simulink model "ac_generator_sysid_R2018a"  (R2018a)
settings: Solver=ode15s  StartTime=0.0  StopTime=12  MaxStep=1e-3  RelTol=1e-3
values from neighbouring files (symbols this model uses):
  f_gen = (1-eff)*P/w_g/w_g    (= 4.2217159851)    [ac_generator_parameters.m]
  h = 0.2    [Apollo_LM_design_discrete_observer.m]    (also in Apollo_LM_design_observer.m = 0.25)
  J_gen = 150    [ac_generator_parameters.m]
  K_gen = P/w_g/sind(30)    [ac_generator_parameters.m]
  w_g = 60*2*pi    (= 376.991118431)    [ac_generator_parameters.m]
undefined symbols (not defined in the file or in its folder): den, num
settings Model: Creator=kjartan  LastModifiedBy=kjartan
settings DataIOCC: ReturnWorkspaceOutputs=on
settings DebuggingCC: UnconnectedInputMsg=none  UnconnectedOutputMsg=none  UnconnectedLineMsg=none  SFMachineParentedDataDiag=error
settings ModelReferenceCC: EnableRefExpFcnMdlSchedulingChecks=off
settings SFSimCC: SimUseLocalCustomCode=on
settings RTWCC: Description=Generic Real-Time Target  RTWUseLocalCustomCode=on

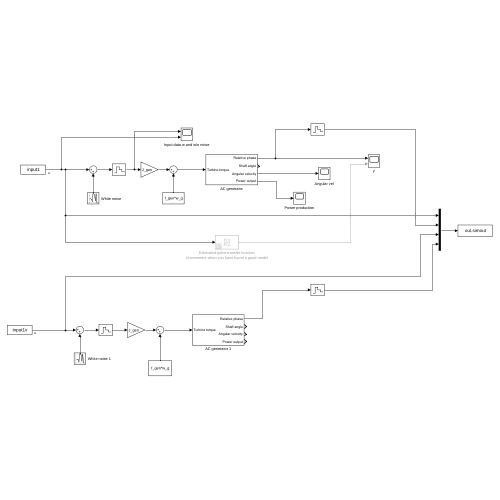
[thumbnail: Simulink's stored preview of the top-level diagram]
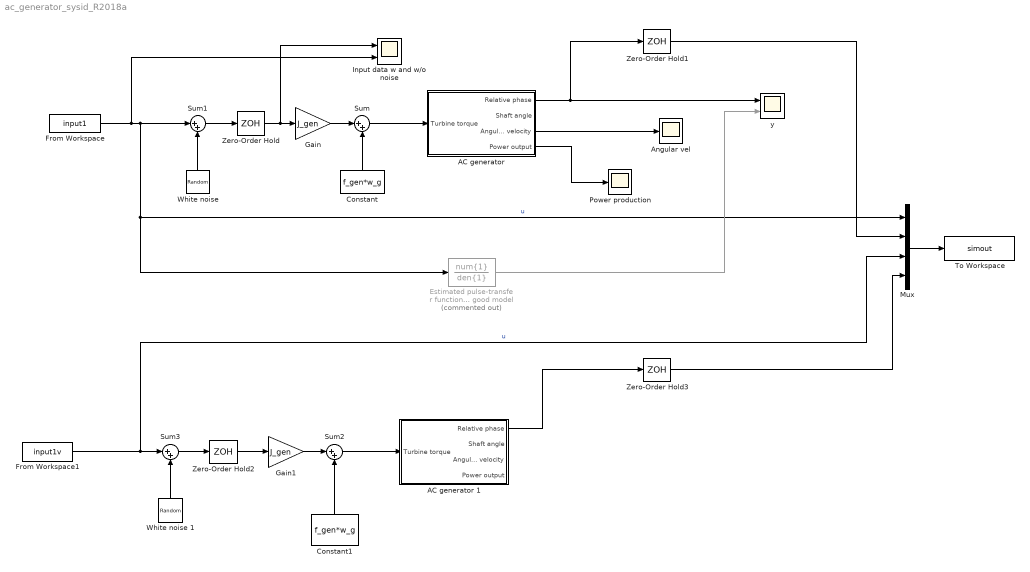
== system ac_generator_sysid_R2018a ==
  AC generator : Subsystem
  AC generator 1 : Subsystem
  Angular vel : Scope
  Constant : Constant  Value=f_gen*w_g
  Constant1 : Constant  Value=f_gen*w_g
  Estimated pulse-transfer function Uncomment when you have found a good model : DiscreteTransferFcn  Commented=on  Numerator=num{1}  Denominator=den{1}  SampleTime=h
  From Workspace : FromWorkspace  VariableName=input1  SampleTime=h
  From Workspace1 : FromWorkspace  VariableName=input1v  SampleTime=h
  Gain : Gain  Gain=J_gen
  Gain1 : Gain  Gain=J_gen
  Input data w and w/o noise : Scope  NumInputPorts=2
  Mux : Mux
  Power production : Scope
  Sum{,1..3} (4 alike) : Sum  Inputs=|++
  To Workspace : ToWorkspace  VariableName=simout  SaveFormat=Timeseries  SampleTime=-1
  White noise : RandomNumber  Variance=0.25  SampleTime=h
  White noise 1 : RandomNumber  Variance=0.25  Seed=9  SampleTime=h
  Zero-Order Hold{,1..3} (4 alike) : ZeroOrderHold  SampleTime=h
  y : Scope  NumInputPorts=2
  wires:
  AC generator/1(Relative phase) -> Zero-Order Hold1/1, y/1
  From Workspace/1 -> Input data w and w/o noise/2, Estimated pulse-transfer function Uncomment when you have found a good model/1, Mux/1, Sum1/1  "u"
  AC generator/3(Angular velocity) -> Angular vel/1
  AC generator/4(Power output) -> Power production/1
  Constant/1 -> Sum/2
  Sum/1 -> AC generator/1(Turbine torque)
  Gain/1 -> Sum/1
  Estimated pulse-transfer function Uncomment when you have found a good model/1 -> y/2
  Zero-Order Hold/1 -> Input data w and w/o noise/1, Gain/1
  Mux/1 -> To Workspace/1
  Zero-Order Hold1/1 -> Mux/2
  Sum1/1 -> Zero-Order Hold/1
  White noise/1 -> Sum1/2
  From Workspace1/1 -> Mux/3, Sum3/1  "u"
  Zero-Order Hold2/1 -> Gain1/1
  Gain1/1 -> Sum2/1
  AC generator 1/1(Relative phase) -> Zero-Order Hold3/1
  Sum3/1 -> Zero-Order Hold2/1
  Constant1/1 -> Sum2/2
  Sum2/1 -> AC generator 1/1(Turbine torque)
  Zero-Order Hold3/1 -> Mux/4
  White noise 1/1 -> Sum3/2

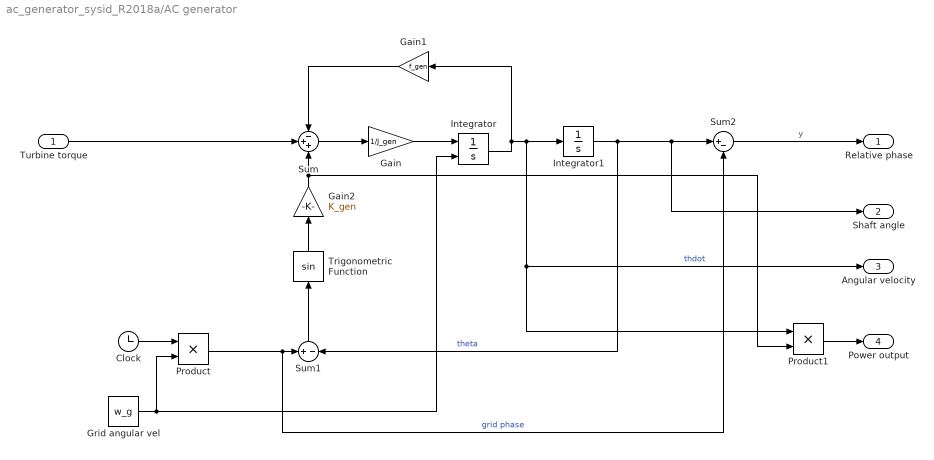
== system ac_generator_sysid_R2018a/AC generator ==
  Turbine torque : Inport
  Clock : Clock
  Gain : Gain  Gain=1/J_gen
  Gain1 : Gain  Gain=f_gen
  Gain2 : Gain  Gain=K_gen
  Grid angular vel : Constant  Value=w_g
  Integrator : Integrator  InitialConditionSource=external
  Integrator1 : Integrator
  Product : Product
  Product1 : Product
  Sum : Sum  Inputs=-++
  Sum1 : Sum  Inputs=+|-
  Sum2 : Sum  Inputs=|+-
  Trigonometric Function : Trigonometry
  Relative phase : Outport
  Shaft angle : Outport  Port=2
  Angular velocity : Outport  Port=3
  Power output : Outport  Port=4
  wires:
  Integrator1/1 -> Shaft angle/1, Sum2/1, Sum1/2  "theta"
  Sum2/1 -> Relative phase/1  "y"
  Gain1/1 -> Sum/1
  Gain2/1 -> Sum/3, Product1/2
  Product/1 -> Sum2/2, Sum1/1  "grid phase"
  Gain/1 -> Integrator/1
  Turbine torque/1 -> Sum/2
  Sum/1 -> Gain/1
  Clock/1 -> Product/1
  Integrator/1 -> Gain1/1, Product1/1, Angular velocity/1, Integrator1/1  "thdot"
  Grid angular vel/1 -> Integrator/2, Product/2
  Product1/1 -> Power output/1
  Sum1/1 -> Trigonometric Function/1
  Trigonometric Function/1 -> Gain2/1

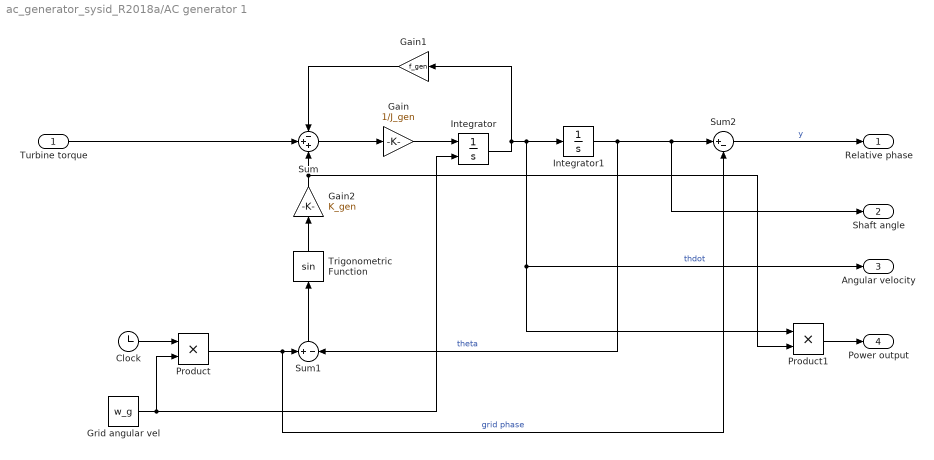
== system ac_generator_sysid_R2018a/AC generator 1 ==
  Turbine torque : Inport
  Clock : Clock
  Gain : Gain  Gain=1/J_gen
  Gain1 : Gain  Gain=f_gen
  Gain2 : Gain  Gain=K_gen
  Grid angular vel : Constant  Value=w_g
  Integrator : Integrator  InitialConditionSource=external
  Integrator1 : Integrator
  Product : Product
  Product1 : Product
  Sum : Sum  Inputs=-++
  Sum1 : Sum  Inputs=+|-
  Sum2 : Sum  Inputs=|+-
  Trigonometric Function : Trigonometry
  Relative phase : Outport
  Shaft angle : Outport  Port=2
  Angular velocity : Outport  Port=3
  Power output : Outport  Port=4
  wires:
  Integrator1/1 -> Shaft angle/1, Sum2/1, Sum1/2  "theta"
  Sum2/1 -> Relative phase/1  "y"
  Gain1/1 -> Sum/1
  Gain2/1 -> Sum/3, Product1/2
  Product/1 -> Sum2/2, Sum1/1  "grid phase"
  Gain/1 -> Integrator/1
  Turbine torque/1 -> Sum/2
  Sum/1 -> Gain/1
  Clock/1 -> Product/1
  Integrator/1 -> Gain1/1, Product1/1, Angular velocity/1, Integrator1/1  "thdot"
  Grid angular vel/1 -> Integrator/2, Product/2
  Product1/1 -> Power output/1
  Sum1/1 -> Trigonometric Function/1
  Trigonometric Function/1 -> Gain2/1
